simulink model "SysConfStateMachTest"  (R2012b)
settings: Solver=ode1  StartTime=0.0  StopTime=Inf  FixedStep=Tsample_simulink  RelTol=1e-3
PostLoadFcn:
  | , if any(exist('dsrtsu_mdlpostloadfcn', 'file') == [2, 3, 6]), try dsrtsu_mdlpostloadfcn('Execute', bdroot); catch fprintf('Error in PostLoadFcn (dsrtsu_mdlpostloadfcn) for model "%s":\n %s\n', bdroot, lasterr); end, end,
values from neighbouring files (symbols this model uses):
  Tsample_simulink = Ts/10    (= 2e-05)    [load_system_parameters.m]
libraries: simulink_extras x2
(part 1 of 9)
settings Model: DSRTSU_INTERNAL_RTI_VER=430  DSRTSU_INTERNAL_RTI_TYPE=rti1103  DSRTSU_INTERNAL_RTIFPGA=20  BufferReuse=off  Creator=Raghav  LastModifiedBy=Raghav
settings OptimizationCC: BlockReduction=off  OptimizeBlockIOStorage=off  BufferReuse=off  ExpressionFolding=off  LocalBlockOutputs=off
settings HardwareCC: ProdIntDivRoundTo=Zero  ProdEndianess=BigEndian  ProdHWDeviceType=Generic->Custom  TargetIntDivRoundTo=Zero  TargetEndianess=BigEndian  TargetHWDeviceType=Generic->Custom
settings RTWCC: SystemTargetFile=rti1103.tlc  MakeCommand=make_rti  TemplateMakefile=rti1103.tmf  Description=dSPACE DS1103 Hardware Platform  ProcessScript=rti1103_make_rtw_hook
settings STFCustomTargetCC: CodeReplacementLibrary=ANSI_C  ParMdlRefBuildCompliant=on  GeneratePreprocessorConditionals=Disable all  MatFileLogging=on  SystemTargetFile=rti1103.tlc
settings GRTTargetCC: CompOptLevelCompliant=off  ConcurrentExecutionCompliant=off  CombineOutputUpdateFcns=off  GRTInterface=on  ExtModeMexFile=noextcomm

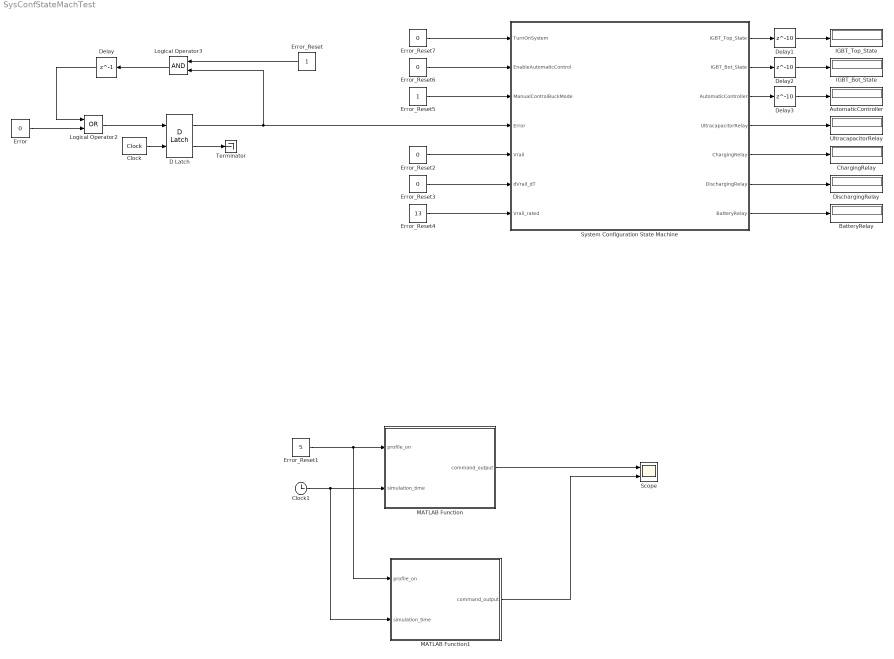
== system SysConfStateMachTest ==
  AutomaticController : Display
  BatteryRelay : Display
  ChargingRelay : Display
  Clock : simulink_extras/Flip Flops/Clock  period=Tsample_simulink*2
  Clock1 : Clock
  D Latch : simulink_extras/Flip Flops/D Latch
  Delay : Delay  DelayLength=1  SampleTime=Tsample_simulink
  Delay1 : Delay  DelayLength=10  SampleTime=Tsample_simulink
  Delay2 : Delay  DelayLength=10  SampleTime=Tsample_simulink
  Delay3 : Delay  DelayLength=10  SampleTime=Tsample_simulink
  DischargingRelay : Display
  Error : Constant  Value=0
  Error_Reset : Constant
  Error_Reset1 : Constant  Value=5
  Error_Reset{2..3,6..7} (4 alike) : Constant  Value=0
  Error_Reset4 : Constant  Value=13
  Error_Reset5 : Constant
  IGBT_Bot_State : Display
  IGBT_Top_State : Display
  Logical Operator2 : Logic  Operator=OR  AllPortsSameDT=off  OutDataTypeStr=boolean
  Logical Operator3 : Logic  AllPortsSameDT=off  OutDataTypeStr=boolean
  MATLAB Function : MATLAB Function  TreatAsAtomicUnit=on
  MATLAB Function1 : MATLAB Function  TreatAsAtomicUnit=on
  Scope : Scope  NumInputPorts=2
      settings: YMin=-1~0  YMax=1~8
  System Configuration State Machine : Stateflow chart  TreatAsAtomicUnit=on
  Terminator : Terminator
  UltracapacitorRelay : Display
  wires:
  System Configuration State Machine/1(IGBT_Top_State) -> Delay1/1
  System Configuration State Machine/2(IGBT_Bot_State) -> Delay2/1
  Clock/1 -> D Latch/2
  D Latch/1 -> Logical Operator3/2, System Configuration State Machine/4(Error)
  Error/1 -> Logical Operator2/2
  Logical Operator2/1 -> D Latch/1
  Logical Operator3/1 -> Delay/1
  Error_Reset/1 -> Logical Operator3/1
  D Latch/2 -> Terminator/1
  Error_Reset2/1 -> System Configuration State Machine/5(Vrail)
  Error_Reset3/1 -> System Configuration State Machine/6(dVrail_dT)
  Error_Reset4/1 -> System Configuration State Machine/7(Vrail_rated)
  Error_Reset5/1 -> System Configuration State Machine/3(ManualControlBuckMode)
  Error_Reset6/1 -> System Configuration State Machine/2(EnableAutomaticControl)
  Error_Reset7/1 -> System Configuration State Machine/1(TurnOnSystem)
  System Configuration State Machine/3(AutomaticController) -> Delay3/1
  System Configuration State Machine/4(UltracapacitorRelay) -> UltracapacitorRelay/1
  System Configuration State Machine/5(ChargingRelay) -> ChargingRelay/1
  System Configuration State Machine/6(DischargingRelay) -> DischargingRelay/1
  System Configuration State Machine/7(BatteryRelay) -> BatteryRelay/1
  Delay/1 -> Logical Operator2/1
  Delay1/1 -> IGBT_Top_State/1
  Delay2/1 -> IGBT_Bot_State/1
  Delay3/1 -> AutomaticController/1
  Error_Reset1/1 -> MATLAB Function1/1(profile_on), MATLAB Function/1(profile_on)
  Clock1/1 -> MATLAB Function1/2(simulation_time), MATLAB Function/2(simulation_time)
  MATLAB Function/1(command_output) -> Scope/1
  MATLAB Function1/1(command_output) -> Scope/2
